simulink model "NXTwaySim"  (R2023a)
settings: Solver=ode4  StartTime=0.0  StopTime=6  FixedStep=0.0001  RelTol=1e-3  EnableMultiTasking=on
undefined symbols (not defined in the file): K, Lc_corrige, R, sigbuilder_block
settings Model: Creator=Lucas  LastModifiedBy=orvik
settings SolverCC: AlgebraicLoopSolver=TrustRegion  SolverResetMethod=Robust
settings DataIOCC: LimitDataPoints=on  SaveFormat=Array  SignalLoggingSaveFormat=ModelDataLogs  ReturnWorkspaceOutputs=off
settings OptimizationCC: ExpressionDepthLimit=2147483647  LifeSpan=inf
settings DebuggingCC: UnderspecifiedInitializationDetection=Classic  MergeDetectMultiDrivingBlocksExec=none  SolverPrmCheckMsg=warning  FcnCallInpInsideContextMsg=warning  UnconnectedInputMsg=warning  UnconnectedOutputMsg=warning  UnconnectedLineMsg=warning  StateNameClashWarn=warning  SFUnexpectedBacktrackingDiag=warning  SFNoUnconditionalDefaultTransitionDiag=warning  SFExecutionAtInitializationDiag=none  ArithmeticOperatorsInVariantConditions=warning
settings HardwareCC: ProdBitPerPointer=32  ProdBitPerSizeT=32  ProdBitPerPtrDiffT=32  ProdLargestAtomicFloat=None  ProdIntDivRoundTo=Undefined  ProdEndianess=Unspecified  ProdWordSize=32  ProdHWDeviceType=32-bit Generic
settings ModelReferenceCC: EnableRefExpFcnMdlSchedulingChecks=on  PropagateSignalLabelsOutOfModel=off
settings SFSimCC: SimUseLocalCustomCode=off  CustomCodeUndefinedFunction=UseInterfaceOnly
settings RTWCC: RTWUseLocalCustomCode=off  DLArmComputeVersion=19.05
settings CodeAppCC: StateflowObjectComments=on
settings GRTTargetCC: TargetLangStandard=C89/C90 (ANSI)  CombineOutputUpdateFcns=off  GRTInterface=on
settings ConfigComp: CovMetricSettings=dw  CovSaveCumulativeToWorkspaceVar=on  CovSaveSingleToWorkspaceVar=on  CovExternalEMLEnable=off

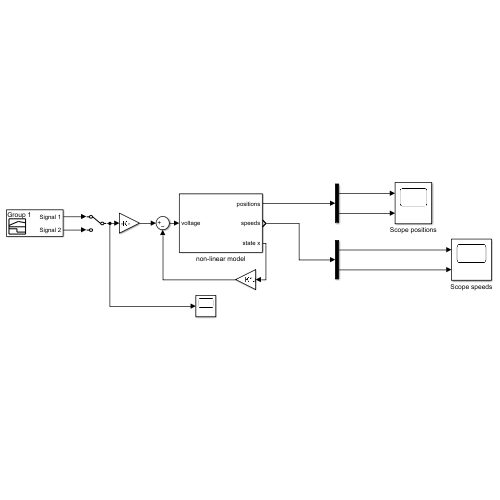
[thumbnail: Simulink's stored preview of the top-level diagram]
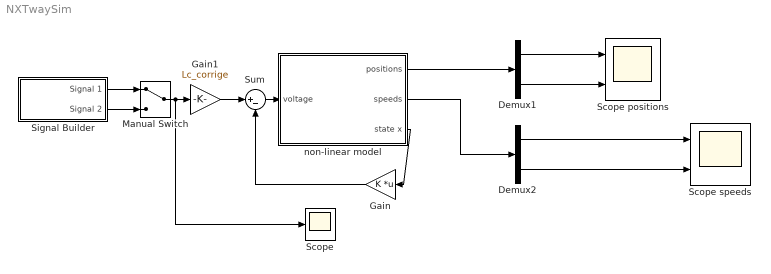
== system NXTwaySim ==
  Demux1 : Demux  Outputs=2
  Demux2 : Demux  Outputs=2
  Gain : Gain  Gain=K  Multiplication=Matrix(K*u)
  Gain1 : Gain  Gain=Lc_corrige
  Manual Switch : ManualSwitch
  Scope : Scope
  Scope positions : Scope  NumInputPorts=2
  Scope speeds : Scope  NumInputPorts=2
  Signal Builder : Subsystem  Tag=STV Subsys  LoadFcn=sigbuilder_block('load');  StartFcn=sigbuilder_block('start');  StopFcn=sigbuilder_block('stop');  ClipboardFcn=sigbuilder_block('clipboard');  mask(Sigbuilder block){tuvar=[0:10]}
      mask help: Simulink:masks:SigbuilderBlock_MD
      mask init:
      | if ~strcmp(get_param(bdroot(gcbh),'SimulationStatus'),'stopped') tuvar = sigbuilder_block('maskInit'); end
      settings: CopyFcn=sigbuilder_block('copy');  DeleteFcn=sigbuilder_block('delete');  ModelCloseFcn=sigbuilder_block('modelClose');  PreSaveFcn=sigbuilder_block('preSave');  PauseFcn=sigbuilder_block('pause');  ContinueFcn=sigbuilder_block('continue');  NameChangeFcn=sigbuilder_block('namechange');  OpenFcn=sigbuilder_block('open',[657 140.25 550.5 399.75 ]);  CloseFcn=sigbuilder_block('close');
      mask Display: plot(0, 0, 100, 100,[2, 2, 32, 32, 2], [68, 8, 8, 68, 68],[32, 2], [38, 38], [32, 19, 2],[53, 60, 44], [32, 17, 17, 2],[16, 16, 31, 31]);txt = getActiveGroup(gcbh);text(2, 100, txt,'verticalAlignment', 'top');
  Sum : Sum  Inputs=|+-
  non-linear model : Subsystem
  wires:
  non-linear model/1(positions) -> Demux1/1
  Demux1/1 -> Scope positions/1
  Demux1/2 -> Scope positions/2
  Demux2/1 -> Scope speeds/1
  Signal Builder/1(Signal 1) -> Manual Switch/1
  Signal Builder/2(Signal 2) -> Manual Switch/2
  non-linear model/2(speeds) -> Demux2/1
  Demux2/2 -> Scope speeds/2
  Sum/1 -> non-linear model/1(voltage)
  non-linear model/3(state x) -> Gain/1
  Gain/1 -> Sum/2
  Manual Switch/1 -> Scope/1, Gain1/1
  Gain1/1 -> Sum/1

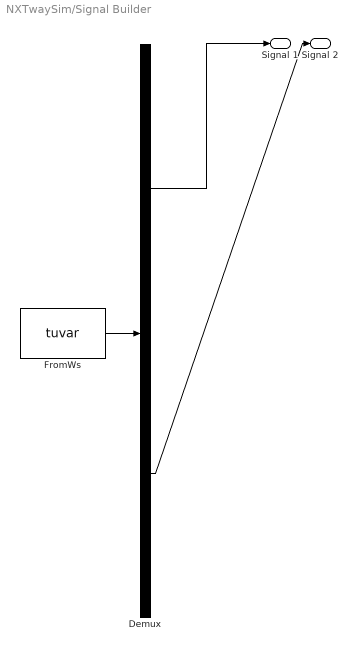
== system NXTwaySim/Signal Builder ==
  Demux : Demux  Tag=STV Demux  Outputs=2
      settings: DisplayOption=none
  FromWs : FromWorkspace  Tag=STV FromWs  VariableName=tuvar
      SigBuilderData=|
      | common.afterFinalStr = 'Extrapolate'
      | common.sampleTime = 0
      | dataSet.timeRange = [0 10]
      | dataSet.name = 'Group 1'
      | sbobj.Groups.Name = 'Group 1'
      | sbobj.Groups.Signals(1).Name = 'Signal 1'
      | sbobj.Groups.Signals(1).XData = [0 1 1 2 2 4 4 5 5 10]
      | sbobj.Groups.Signals(1).YData = [0 0 5 5 0 0 -3 -3 0 0]
      | sbobj.Groups.Signals(2).Name = 'Signal 2'
      | sbobj.Groups.Signals(2).XData = [0 0.125 0.25 0.375 0.5 0.625 0.75 0.875 1 1.125 1.25 1.375 1.5 1.625 1.75 1.875 2 2.125 2.25 2.375 2.5 2.625 2.75 2.875 3 3.125 3.25 3.375 3.5 3.625 3.75 3.875 4 4.125 4.25 4.375 4.5 4.625 4.75 4.875 5 5.125 5.25 5.375 5.5 5.625 5.75 5.875 6 6.125 6.25 6.375 6.5 6.625 6.75 6.875 7 7.125 7.25 7.375 7.5 7.625 7.75 7.875 8 8.125 8.25 8.375 8.5 8.625 8.75 8.875 9 9.125 9.25 9.375 9.5 9.625 9.75 9.875 10]
      | sbobj.Groups.Signals(2).YData = [0 0.707106781187 1 0.707106781187 1.22464679915e-16 -0.707106781187 -1 -0.707106781187 0 0.707106781187 1 0.707106781187 1.22464679915e-16 -0.707106781187 -1 -0.707106781187 0 0.707106781187 1 0.707106781187 1.22464679915e-16 -0.707106781187 -1 -0.707106781187 0 0.707106781187 1 0.707106781187 1.22464679915e-16 -0.707106781187 -1 -0.707106781187 0 0.707106781187 1 0.707106781187 1.22464679915e-16 -0.707106781187 -1 -0.707106781187 0 0.707106781187 1 0.707106781187 1.22464679915e-16 -0.707106781187 -1 -0.707106781187 0 0.707106781187 1 0.707106781187 1.22464679915e-16 -0.707106781187 -1 -0.707106781187 0 0.707106781187 1 0.707106781187 1.22464679915e-16 -0.707106781187 -1 -0.707106781187 0 0.707106781187 1 0.707106781187 1.22464679915e-16 -0.707106781187 -1 -0.707106781187 0 0.707106781187 1 0.707106781187 1.22464679915e-16 -0.707106781187 -1 -0.707106781187 0]
  Signal 1 : Outport  Tag=STV Outport
  Signal 2 : Outport  Tag=STV Outport  Port=2
  wires:
  Demux/1 -> Signal 1/1
  FromWs/1 -> Demux/1
  Demux/2 -> Signal 2/1

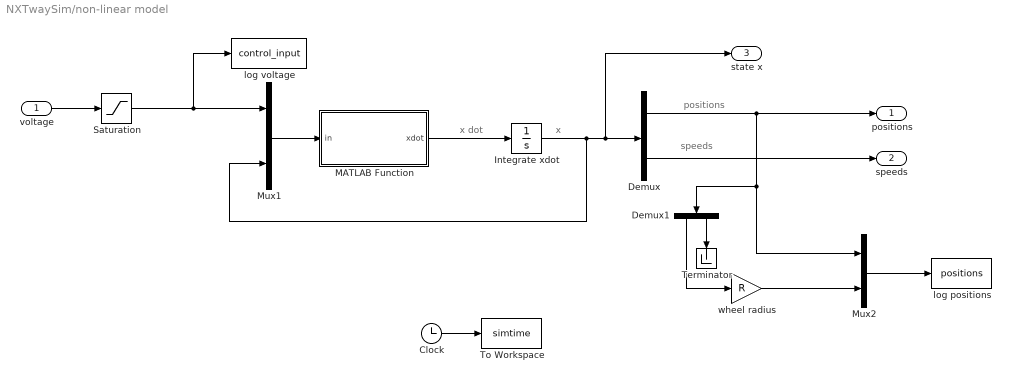
== system NXTwaySim/non-linear model ==
  note: speeds
  note: x dot
  note: x
  note: positions
  voltage : Inport
  Clock : Clock
  Demux : Demux  Outputs=2
  Demux1 : Demux  Outputs=2
  Integrate xdot : Integrator  InitialCondition=[0;0;0;0]
  MATLAB Function : MATLAB Function  TreatAsAtomicUnit=on
  Mux1 : Mux  Inputs=2
  Mux2 : Mux  Inputs=2
  Saturation : Saturate  UpperLimit=8  LowerLimit=-8
  Terminator : Terminator
  To Workspace : ToWorkspace  VariableName=simtime  SampleTime=-1
      settings: Decimation=100
  log positions : ToWorkspace  VariableName=positions  SampleTime=-1
      settings: Decimation=100
  log voltage : ToWorkspace  VariableName=control_input  SampleTime=-1
  wheel radius : Gain  Gain=R
  positions : Outport
  speeds : Outport  Port=2
  state x : Outport  Port=3
  wires:
  Mux1/1 -> MATLAB Function/1(in)
  MATLAB Function/1(xdot) -> Integrate xdot/1
  Demux/1 -> Mux2/1, Demux1/1, positions/1
  voltage/1 -> Saturation/1
  Demux/2 -> speeds/1
  Demux1/2 -> Terminator/1
  Demux1/1 -> wheel radius/1
  Mux2/1 -> log positions/1
  wheel radius/1 -> Mux2/2
  Integrate xdot/1 -> Mux1/2, state x/1, Demux/1
  Clock/1 -> To Workspace/1
  Saturation/1 -> Mux1/1, log voltage/1

== matlab function NXTwaySim/non-linear model/MATLAB Function ==
  data: in input; xdot output
function xdot =  compute_xdot(in)
%
% This function computes the x dot vector of the system (state derivative). It is used in
% the simulation simulink file to run the dynamical model of the
% gyropode.

% system parameters (defined in initialisation.m)
g = 9.80665;                    
m = 0.03;						
R = 0.042;						
Jw = m * R^2 / 2;				
M = 0.67;						
W = 0.165;						
D = 0.05;						
H = 0.152;						
L = H / 2;						
Jpsi = M * L^2 / 3;				
fm = 0.0022;					
fw = 0;								
Jm = 1e-5;						
Rm = 6.8327;					
Kb = 0.468;						
Kt = 0.3047;					
n = 1;							

% input arguments
% control signal
u = in(1);         % input voltage for the motors
% position vector
theta = in(2);       % angular position of the wheel
psi = in(3);       % angular position of the gyropode
% speed vector
dtheta = in(4);       % angular speed of the wheel
dpsi = in(5);       % angular speed of the gyropode



% computes the value of the x dot vector (state derivative)
i = 1/Rm * ( u + Kb*(dpsi-dtheta) );
Ftheta = 2*( n*Kt*i + fm*(dpsi-dtheta) - fw*dtheta );
%Ftheta = n*Kt*i + fm*(dpsi-dtheta) - fw*dtheta;
Fpsi = -2*n*Kt*i - 2*fm*(dpsi-dtheta);
%Fpsi = -n*Kt*i - fm*(dpsi-dtheta);
M1 = [ ((2*m+M)*R^2+2*Jw+2*n^2*Jm)  (M*L*R*cos(psi)-2*n^2*Jm) ;
       (M*L*R*cos(psi)-2*n^2*Jm)    (M*L^2+Jpsi+2*n^2*Jm) ];
M2 = [ Ftheta+M*L*R*dpsi^2*sin(psi);
       Fpsi+M*g*L*sin(psi)];
var = M1\M2;

xdot1 = dtheta;
xdot2 = dpsi;
xdot3 = var(1);
xdot4 = var(2);

xdot = [xdot1;xdot2;xdot3;xdot4];
